simulink library "customlib"  (R2015b)
settings: Solver=ode45  StartTime=0.0  StopTime=10.0  RelTol=1e-3
libraries: dspsigops x5
settings Model: Creator=amatsumo  LastModifiedBy=amatsumo
settings DataIOCC: SaveFormat=Array  SignalLoggingSaveFormat=ModelDataLogs
settings OptimizationCC: ExpressionDepthLimit=2147483647
settings DebuggingCC: UnderspecifiedInitializationDetection=Classic  MergeDetectMultiDrivingBlocksExec=none  SolverPrmCheckMsg=warning  FcnCallInpInsideContextMsg=UseLocalSettings  StateNameClashWarn=warning  StrictBusMsg=Warning
settings HardwareCC: ProdBitPerPointer=32  ProdLargestAtomicFloat=None  ProdIntDivRoundTo=Undefined  ProdEndianess=Unspecified  ProdWordSize=32  ProdHWDeviceType=32-bit Generic
settings GRTTargetCC: GeneratePreprocessorConditionals=Disable all  CombineOutputUpdateFcns=off  GRTInterface=on
settings ConfigComp: CovModelRefEnable=Off  CovSFcnEnable=off

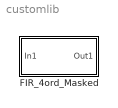
== system customlib ==
  FIR_4ord_Masked : Subsystem  mask(4次FIRフィルタ){H=[1 0 3 0 1]/4, pipeline=0}
      mask prompts: H "Coefficients(5個)"; pipeline "Pipeline Level"
      mask help: フィルタの係数（5個）と積和演算後のパイプラインレベル（FF数）を設定して下さい。
      mask init:
      | str1 = ['H = ', num2str(H)];
      | str2 = ['Pipeline Level = ', num2str(pipeline)];
      | strvcat(str1,str2)
      mask Help: FIRフィルタのヘルプドキュメントを記述します。

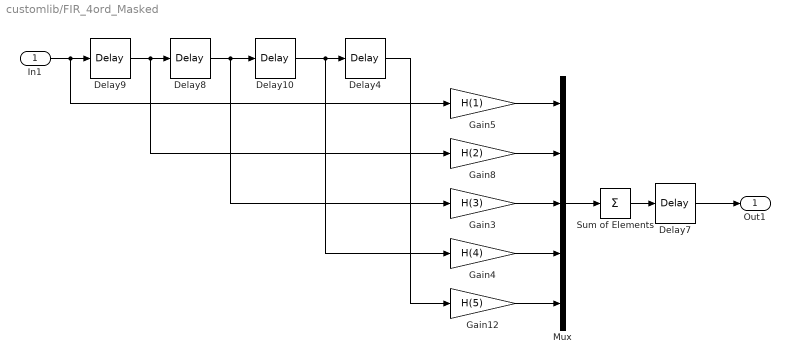
== system customlib/FIR_4ord_Masked ==
  In1 : Inport
  Delay{4,8..10} (4 alike) : dspsigops/Delay  InputProcessing=Inherited (this choice will be removed - see release notes)  dly_unit=Samples  delay=1  ic_detail=off  dif_ic_for_ch=off  dif_ic_for_dly=off  ic=0  reset_popup=None
  Delay7 : dspsigops/Delay  InputProcessing=Inherited (this choice will be removed - see release notes)  dly_unit=Samples  delay=pipeline  ic_detail=off  dif_ic_for_ch=off  dif_ic_for_dly=off  ic=0  reset_popup=None
  Gain12 : Gain  Gain=H(5)  RndMeth=Nearest  OutDataTypeStr=Inherit: Same as input
  Gain3 : Gain  Gain=H(3)  RndMeth=Nearest  OutDataTypeStr=Inherit: Same as input
  Gain4 : Gain  Gain=H(4)  RndMeth=Nearest  OutDataTypeStr=Inherit: Same as input
  Gain5 : Gain  Gain=H(1)  RndMeth=Nearest  OutDataTypeStr=Inherit: Same as input
  Gain8 : Gain  Gain=H(2)  RndMeth=Nearest  OutDataTypeStr=Inherit: Same as input
  Mux : Mux  Inputs=5
  Sum of Elements : Sum  Inputs=+  RndMeth=Nearest
  Out1 : Outport
  wires:
  Delay7/1 -> Out1/1
  In1/1 -> Delay9/1, Gain5/1
  Delay10/1 -> Gain4/1, Delay4/1
  Delay9/1 -> Gain8/1, Delay8/1
  Delay8/1 -> Gain3/1, Delay10/1
  Mux/1 -> Sum of Elements/1
  Delay4/1 -> Gain12/1
  Gain5/1 -> Mux/1
  Gain8/1 -> Mux/2
  Gain3/1 -> Mux/3
  Gain4/1 -> Mux/4
  Gain12/1 -> Mux/5
  Sum of Elements/1 -> Delay7/1
